simulink model "Study on wave sampling system using MATLAB software"  (R2016a)
settings: Solver=VariableStepAuto  StartTime=0.0  StopTime=8  RelTol=1e-3
settings Model: Creator=ahpar  LastModifiedBy=ahpar

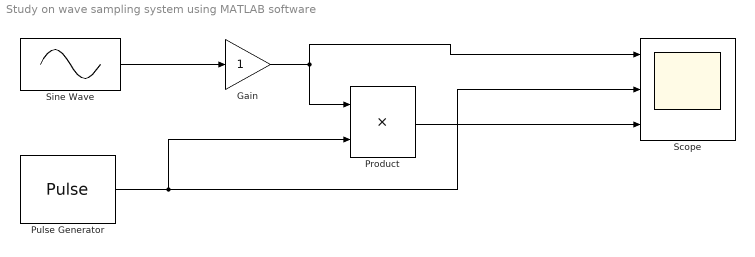
== system Study on wave sampling system using MATLAB software ==
  Gain : Gain
  Product : Product
  Pulse Generator : DiscretePulseGenerator  PulseType=Time based  Period=0.01
  Scope : Scope  NumInputPorts=3
  Sine Wave : Sin  SampleTime=0
  wires:
  Pulse Generator/1 -> Scope/2, Product/2
  Product/1 -> Scope/3
  Sine Wave/1 -> Gain/1
  Gain/1 -> Scope/1, Product/1
